simulink model "Sensor"  (R2022b)
settings: configuration reference "TmVcThermal_Configuration_sub" (kept outside this file)
undefined symbols (not defined in the file): cClCddSensor_t_u8AQSErrorConfirm, cClCddSensor_t_u8AQSErrorRelieve, cClCddSensor_Te_s32HvacEvapSensorOpenOrShortGnd, cClCddSensor_Te_s32HvacEvapSensorShortBatt, cClCddSensor_Te_s32HvacHexSensorOpenOrShortGnd, cClCddSensor_Te_s32HvacHexSensorShortBatt, cClCddSensor_Te_s32HvacIncarSensorOpenOrShortGnd, cClCddSensor_Te_s32HvacIncarSensorShortBatt, cClCddSensor_X_u8AQSErrorShape, cClCddSensor_X_u8AQSErrorShapeDevia, tClCddSensor_Te_s32EvapRtValue, tClCddSensor_Te_s32EvapRtValue_X, tClCddSensor_Te_s32HexRtValue, tClCddSensor_Te_s32HexRtValue_X, tClCddSensor_Te_s32IncarRtValue, tClCddSensor_Te_s32IncarRtValue_X
libraries: PCMULib x3, simulink x2
settings Model: PacingRate=0.500000  Creator=blue.ge  LastModifiedBy=blue.ge
settings ConfigSetRef: SourceName=TmVcThermal_Configuration_sub  SourceLocation=Base Workspace

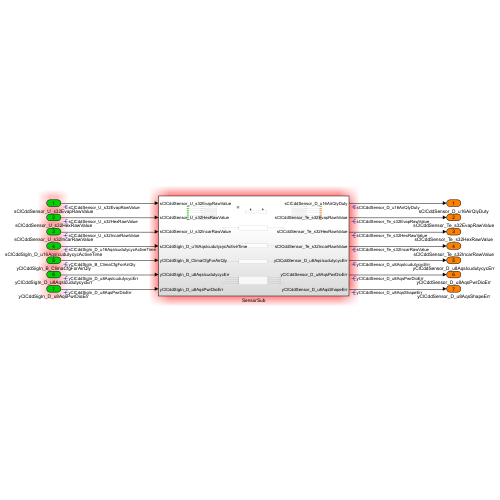
[thumbnail: Simulink's stored preview of the top-level diagram]
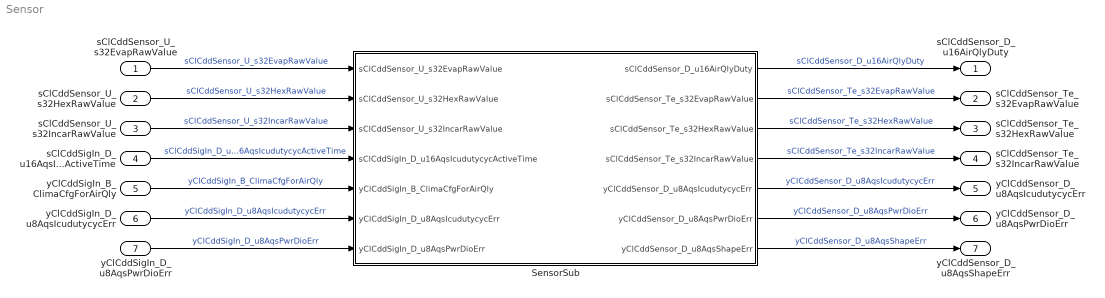
== system Sensor ==
  sClCddSensor_U_s32EvapRawValue : Inport  OutDataTypeStr=single
  sClCddSensor_U_s32HexRawValue : Inport  Port=2  OutDataTypeStr=single
  sClCddSensor_U_s32IncarRawValue : Inport  Port=3  OutDataTypeStr=single
  sClCddSigIn_D_u16AqsIcudutycycActiveTime : Inport  Port=4  OutDataTypeStr=uint16
  yClCddSigIn_B_ClimaCfgForAirQly : Inport  Port=5  OutDataTypeStr=boolean
  yClCddSigIn_D_u8AqsIcudutycycErr : Inport  Port=6  OutDataTypeStr=uint8
  yClCddSigIn_D_u8AqsPwrDioErr : Inport  Port=7  OutDataTypeStr=uint8
  SensorSub : Subsystem
  sClCddSensor_D_u16AirQlyDuty : Outport  OutDataTypeStr=uint16
  sClCddSensor_Te_s32EvapRawValue : Outport  Port=2  OutDataTypeStr=single
  sClCddSensor_Te_s32HexRawValue : Outport  Port=3  OutDataTypeStr=single
  sClCddSensor_Te_s32IncarRawValue : Outport  Port=4  OutDataTypeStr=single
  yClCddSensor_D_u8AqsIcudutycycErr : Outport  Port=5  OutDataTypeStr=uint8
  yClCddSensor_D_u8AqsPwrDioErr : Outport  Port=6  OutDataTypeStr=uint8
  yClCddSensor_D_u8AqsShapeErr : Outport  Port=7  OutDataTypeStr=uint8
  wires:
  SensorSub/5(yClCddSensor_D_u8AqsIcudutycycErr) -> yClCddSensor_D_u8AqsIcudutycycErr/1  "yClCddSensor_D_u8AqsIcudutycycErr"
  SensorSub/4(sClCddSensor_Te_s32IncarRawValue) -> sClCddSensor_Te_s32IncarRawValue/1  "sClCddSensor_Te_s32IncarRawValue"
  SensorSub/7(yClCddSensor_D_u8AqsShapeErr) -> yClCddSensor_D_u8AqsShapeErr/1  "yClCddSensor_D_u8AqsShapeErr"
  SensorSub/2(sClCddSensor_Te_s32EvapRawValue) -> sClCddSensor_Te_s32EvapRawValue/1  "sClCddSensor_Te_s32EvapRawValue"
  SensorSub/6(yClCddSensor_D_u8AqsPwrDioErr) -> yClCddSensor_D_u8AqsPwrDioErr/1  "yClCddSensor_D_u8AqsPwrDioErr"
  SensorSub/1(sClCddSensor_D_u16AirQlyDuty) -> sClCddSensor_D_u16AirQlyDuty/1  "sClCddSensor_D_u16AirQlyDuty"
  yClCddSigIn_D_u8AqsIcudutycycErr/1 -> SensorSub/6(yClCddSigIn_D_u8AqsIcudutycycErr)  "yClCddSigIn_D_u8AqsIcudutycycErr"
  sClCddSensor_U_s32EvapRawValue/1 -> SensorSub/1(sClCddSensor_U_s32EvapRawValue)  "sClCddSensor_U_s32EvapRawValue"
  sClCddSensor_U_s32IncarRawValue/1 -> SensorSub/3(sClCddSensor_U_s32IncarRawValue)  "sClCddSensor_U_s32IncarRawValue"
  yClCddSigIn_D_u8AqsPwrDioErr/1 -> SensorSub/7(yClCddSigIn_D_u8AqsPwrDioErr)  "yClCddSigIn_D_u8AqsPwrDioErr"
  sClCddSensor_U_s32HexRawValue/1 -> SensorSub/2(sClCddSensor_U_s32HexRawValue)  "sClCddSensor_U_s32HexRawValue"
  SensorSub/3(sClCddSensor_Te_s32HexRawValue) -> sClCddSensor_Te_s32HexRawValue/1  "sClCddSensor_Te_s32HexRawValue"
  yClCddSigIn_B_ClimaCfgForAirQly/1 -> SensorSub/5(yClCddSigIn_B_ClimaCfgForAirQly)  "yClCddSigIn_B_ClimaCfgForAirQly"
  sClCddSigIn_D_u16AqsIcudutycycActiveTime/1 -> SensorSub/4(sClCddSigIn_D_u16AqsIcudutycycActiveTime)  "sClCddSigIn_D_u16AqsIcudutycycActiveTime"

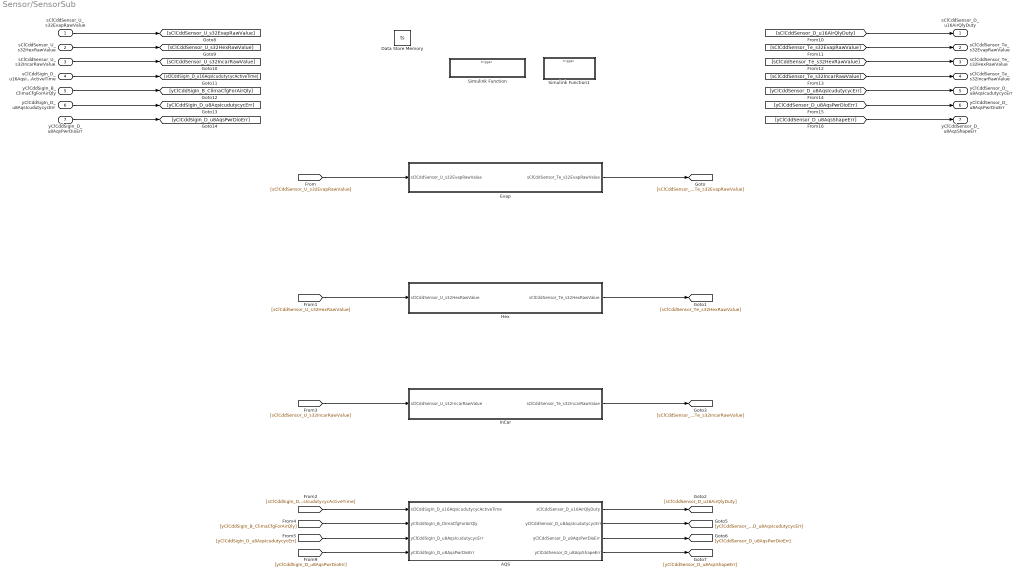
== system Sensor/SensorSub ==
  sClCddSensor_U_s32EvapRawValue : Inport  OutDataTypeStr=single
  sClCddSensor_U_s32HexRawValue : Inport  Port=2  OutDataTypeStr=single
  sClCddSensor_U_s32IncarRawValue : Inport  Port=3  OutDataTypeStr=single
  sClCddSigIn_D_u16AqsIcudutycycActiveTime : Inport  Port=4  OutDataTypeStr=uint16
  yClCddSigIn_B_ClimaCfgForAirQly : Inport  Port=5  OutDataTypeStr=boolean
  yClCddSigIn_D_u8AqsIcudutycycErr : Inport  Port=6  OutDataTypeStr=uint8
  yClCddSigIn_D_u8AqsPwrDioErr : Inport  Port=7  OutDataTypeStr=uint8
  AQS : Subsystem
  Data Store Memory : DataStoreMemory  DataStoreName=ts  ReadBeforeWriteMsg=warning  WriteAfterWriteMsg=warning  WriteAfterReadMsg=warning  InitialValue=0.05  ShowAdditionalParam=off  OutDataTypeStr=single
      settings: CopyFcn=set_param(gcbh,'ShowName','off');
  Evap : Subsystem
  Hex : Subsystem
  InCar : Subsystem
  Simulink Function : Subsystem  TreatAsAtomicUnit=on
  Simulink Function1 : Subsystem  TreatAsAtomicUnit=on
  sClCddSensor_D_u16AirQlyDuty : Outport  OutDataTypeStr=uint16
  sClCddSensor_Te_s32EvapRawValue : Outport  Port=2  OutDataTypeStr=single
  sClCddSensor_Te_s32HexRawValue : Outport  Port=3  OutDataTypeStr=single
  sClCddSensor_Te_s32IncarRawValue : Outport  Port=4  OutDataTypeStr=single
  yClCddSensor_D_u8AqsIcudutycycErr : Outport  Port=5  OutDataTypeStr=uint8
  yClCddSensor_D_u8AqsPwrDioErr : Outport  Port=6  OutDataTypeStr=uint8
  yClCddSensor_D_u8AqsShapeErr : Outport  Port=7  OutDataTypeStr=uint8
  wires:
  [sClCddSensor_U_s32EvapRawValue] -> Evap/1(sClCddSensor_U_s32EvapRawValue)
  Evap/1(sClCddSensor_Te_s32EvapRawValue) -> [sClCddSensor_Te_s32EvapRawValue]
  [sClCddSensor_U_s32HexRawValue] -> Hex/1(sClCddSensor_U_s32HexRawValue)
  Hex/1(sClCddSensor_Te_s32HexRawValue) -> [sClCddSensor_Te_s32HexRawValue]
  [sClCddSensor_U_s32IncarRawValue] -> InCar/1(sClCddSensor_U_s32IncarRawValue)
  InCar/1(sClCddSensor_Te_s32IncarRawValue) -> [sClCddSensor_Te_s32IncarRawValue]
  [sClCddSigIn_D_u16AqsIcudutycycActiveTime] -> AQS/1(sClCddSigIn_D_u16AqsIcudutycycActiveTime)
  [yClCddSigIn_B_ClimaCfgForAirQly] -> AQS/2(yClCddSigIn_B_ClimaCfgForAirQly)
  [yClCddSigIn_D_u8AqsIcudutycycErr] -> AQS/3(yClCddSigIn_D_u8AqsIcudutycycErr)
  [yClCddSigIn_D_u8AqsPwrDioErr] -> AQS/4(yClCddSigIn_D_u8AqsPwrDioErr)
  AQS/1(sClCddSensor_D_u16AirQlyDuty) -> [sClCddSensor_D_u16AirQlyDuty]
  AQS/2(yClCddSensor_D_u8AqsIcudutycycErr) -> [yClCddSensor_D_u8AqsIcudutycycErr]
  AQS/3(yClCddSensor_D_u8AqsPwrDioErr) -> [yClCddSensor_D_u8AqsPwrDioErr]
  AQS/4(yClCddSensor_D_u8AqsShapeErr) -> [yClCddSensor_D_u8AqsShapeErr]
  sClCddSensor_U_s32EvapRawValue/1 -> [sClCddSensor_U_s32EvapRawValue]
  sClCddSensor_U_s32HexRawValue/1 -> [sClCddSensor_U_s32HexRawValue]
  sClCddSensor_U_s32IncarRawValue/1 -> [sClCddSensor_U_s32IncarRawValue]
  sClCddSigIn_D_u16AqsIcudutycycActiveTime/1 -> [sClCddSigIn_D_u16AqsIcudutycycActiveTime]
  yClCddSigIn_B_ClimaCfgForAirQly/1 -> [yClCddSigIn_B_ClimaCfgForAirQly]
  yClCddSigIn_D_u8AqsIcudutycycErr/1 -> [yClCddSigIn_D_u8AqsIcudutycycErr]
  yClCddSigIn_D_u8AqsPwrDioErr/1 -> [yClCddSigIn_D_u8AqsPwrDioErr]
  [sClCddSensor_D_u16AirQlyDuty] -> sClCddSensor_D_u16AirQlyDuty/1
  [sClCddSensor_Te_s32EvapRawValue] -> sClCddSensor_Te_s32EvapRawValue/1
  [sClCddSensor_Te_s32HexRawValue] -> sClCddSensor_Te_s32HexRawValue/1
  [sClCddSensor_Te_s32IncarRawValue] -> sClCddSensor_Te_s32IncarRawValue/1
  [yClCddSensor_D_u8AqsIcudutycycErr] -> yClCddSensor_D_u8AqsIcudutycycErr/1
  [yClCddSensor_D_u8AqsPwrDioErr] -> yClCddSensor_D_u8AqsPwrDioErr/1
  [yClCddSensor_D_u8AqsShapeErr] -> yClCddSensor_D_u8AqsShapeErr/1

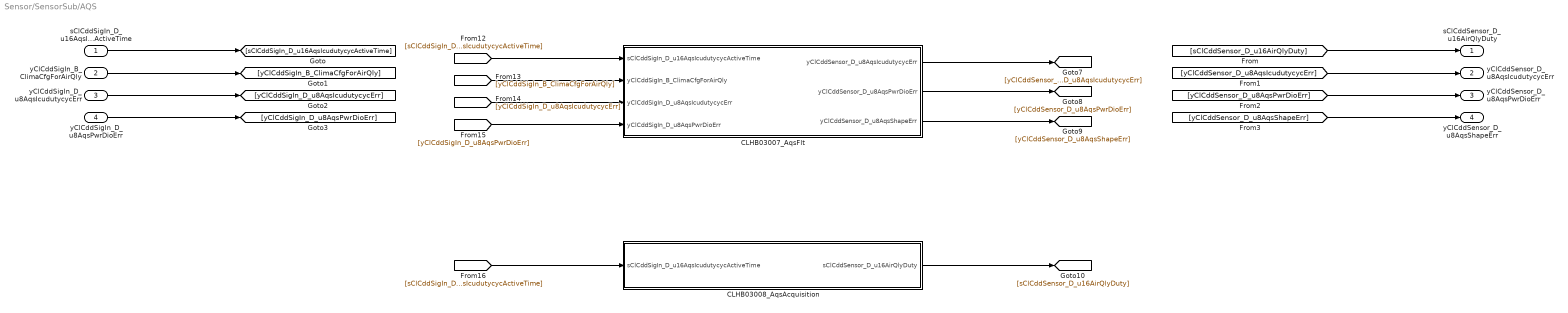
== system Sensor/SensorSub/AQS ==
  sClCddSigIn_D_u16AqsIcudutycycActiveTime : Inport  OutDataTypeStr=uint16
  yClCddSigIn_B_ClimaCfgForAirQly : Inport  Port=2  OutDataTypeStr=boolean
  yClCddSigIn_D_u8AqsIcudutycycErr : Inport  Port=3  OutDataTypeStr=uint8
  yClCddSigIn_D_u8AqsPwrDioErr : Inport  Port=4  OutDataTypeStr=uint8
  CLHB03007_AqsFlt : Subsystem
  CLHB03008_AqsAcquisition : Subsystem
  sClCddSensor_D_u16AirQlyDuty : Outport  OutDataTypeStr=uint16
  yClCddSensor_D_u8AqsIcudutycycErr : Outport  Port=2  OutDataTypeStr=uint8
  yClCddSensor_D_u8AqsPwrDioErr : Outport  Port=3  OutDataTypeStr=uint8
  yClCddSensor_D_u8AqsShapeErr : Outport  Port=4  OutDataTypeStr=uint8
  wires:
  [yClCddSigIn_D_u8AqsIcudutycycErr] -> CLHB03007_AqsFlt/3(yClCddSigIn_D_u8AqsIcudutycycErr)
  [sClCddSigIn_D_u16AqsIcudutycycActiveTime] -> CLHB03008_AqsAcquisition/1(sClCddSigIn_D_u16AqsIcudutycycActiveTime)
  CLHB03007_AqsFlt/2(yClCddSensor_D_u8AqsPwrDioErr) -> [yClCddSensor_D_u8AqsPwrDioErr]
  CLHB03007_AqsFlt/1(yClCddSensor_D_u8AqsIcudutycycErr) -> [yClCddSensor_D_u8AqsIcudutycycErr]
  [sClCddSigIn_D_u16AqsIcudutycycActiveTime] -> CLHB03007_AqsFlt/1(sClCddSigIn_D_u16AqsIcudutycycActiveTime)
  CLHB03008_AqsAcquisition/1(sClCddSensor_D_u16AirQlyDuty) -> [sClCddSensor_D_u16AirQlyDuty]
  [yClCddSigIn_B_ClimaCfgForAirQly] -> CLHB03007_AqsFlt/2(yClCddSigIn_B_ClimaCfgForAirQly)
  CLHB03007_AqsFlt/3(yClCddSensor_D_u8AqsShapeErr) -> [yClCddSensor_D_u8AqsShapeErr]
  [yClCddSigIn_D_u8AqsPwrDioErr] -> CLHB03007_AqsFlt/4(yClCddSigIn_D_u8AqsPwrDioErr)
  sClCddSigIn_D_u16AqsIcudutycycActiveTime/1 -> [sClCddSigIn_D_u16AqsIcudutycycActiveTime]
  yClCddSigIn_B_ClimaCfgForAirQly/1 -> [yClCddSigIn_B_ClimaCfgForAirQly]
  yClCddSigIn_D_u8AqsIcudutycycErr/1 -> [yClCddSigIn_D_u8AqsIcudutycycErr]
  yClCddSigIn_D_u8AqsPwrDioErr/1 -> [yClCddSigIn_D_u8AqsPwrDioErr]
  [sClCddSensor_D_u16AirQlyDuty] -> sClCddSensor_D_u16AirQlyDuty/1
  [yClCddSensor_D_u8AqsIcudutycycErr] -> yClCddSensor_D_u8AqsIcudutycycErr/1
  [yClCddSensor_D_u8AqsPwrDioErr] -> yClCddSensor_D_u8AqsPwrDioErr/1
  [yClCddSensor_D_u8AqsShapeErr] -> yClCddSensor_D_u8AqsShapeErr/1

== system Sensor/SensorSub/Evap ==
  sClCddSensor_U_s32EvapRawValue : Inport  OutDataTypeStr=single
  CLHB03002_EvapChange : Subsystem
  CLHB03002_EvapFlt : Subsystem
  sClCddSensor_Te_s32EvapRawValue : Outport  OutDataTypeStr=single
  wires:
  [sClCddSensor_U_s32EvapRawValue] -> CLHB03002_EvapFlt/1(sClCddSensor_U_s32EvapRawValue)
  [sClCddSensor_D_u8HvacEvapSensorErr] -> CLHB03002_EvapChange/2(sClCddSensor_D_u8HvacEvapSensorErr)
  CLHB03002_EvapChange/1(sClCddSensor_Te_s32EvapRawValue) -> [sClCddSensor_Te_s32EvapRawValue]
  CLHB03002_EvapFlt/1(sClCddSensor_D_u8HvacEvapSensorErr) -> [sClCddSensor_D_u8HvacEvapSensorErr]
  [sClCddSensor_U_s32EvapRawValue] -> CLHB03002_EvapChange/1(sClCddSensor_U_s32EvapRawValue)
  sClCddSensor_U_s32EvapRawValue/1 -> [sClCddSensor_U_s32EvapRawValue]
  [sClCddSensor_Te_s32EvapRawValue] -> sClCddSensor_Te_s32EvapRawValue/1

== system Sensor/SensorSub/Hex ==
  sClCddSensor_U_s32HexRawValue : Inport  OutDataTypeStr=single
  CLHB03003_HexFlt : Subsystem
  CLHB03004_HexChange : Subsystem
  sClCddSensor_Te_s32HexRawValue : Outport  OutDataTypeStr=single
  wires:
  [sClCddSensor_U_s32HexRawValue] -> CLHB03003_HexFlt/1(sClCddSensor_U_s32HexRawValue)
  CLHB03003_HexFlt/1(sClCddSensor_D_u8HvacHexSensorErr) -> [sClCddSensor_D_u8HvacHexSensorErr]
  [sClCddSensor_U_s32HexRawValue] -> CLHB03004_HexChange/1("sClCddSensor_U_s32HexRawValue ")
  [sClCddSensor_D_u8HvacHexSensorErr] -> CLHB03004_HexChange/2("sClCddSensor_D_u8HvacHexSensorErr ")
  CLHB03004_HexChange/1("sClCddSensor_Te_s32HexRawValue ") -> [sClCddSensor_Te_s32HexRawValue]
  sClCddSensor_U_s32HexRawValue/1 -> [sClCddSensor_U_s32HexRawValue]
  [sClCddSensor_Te_s32HexRawValue] -> sClCddSensor_Te_s32HexRawValue/1

== system Sensor/SensorSub/InCar ==
  sClCddSensor_U_s32IncarRawValue : Inport  OutDataTypeStr=single
  CLHB03005_InCarFlt : Subsystem
  CLHB03006_InCarChange : Subsystem
  sClCddSensor_Te_s32IncarRawValue : Outport  OutDataTypeStr=single
  wires:
  CLHB03006_InCarChange/1(sClCddSensor_Te_s32IncarRawValue) -> [sClCddSensor_Te_s32IncarRawValue]
  [sClCddSensor_U_s32IncarRawValue] -> CLHB03005_InCarFlt/1(sClCddSensor_U_s32IncarRawValue)
  CLHB03005_InCarFlt/1(sClCddSensor_D_u8HvacIncarSensorErr) -> [sClCddSensor_D_u8HvacIncarSensorErr]
  [sClCddSensor_D_u8HvacIncarSensorErr] -> CLHB03006_InCarChange/1(sClCddSensor_D_u8HvacIncarSensorErr)
  [sClCddSensor_U_s32IncarRawValue] -> CLHB03006_InCarChange/2(sClCddSensor_U_s32IncarRawValue)
  sClCddSensor_U_s32IncarRawValue/1 -> [sClCddSensor_U_s32IncarRawValue]
  [sClCddSensor_Te_s32IncarRawValue] -> sClCddSensor_Te_s32IncarRawValue/1

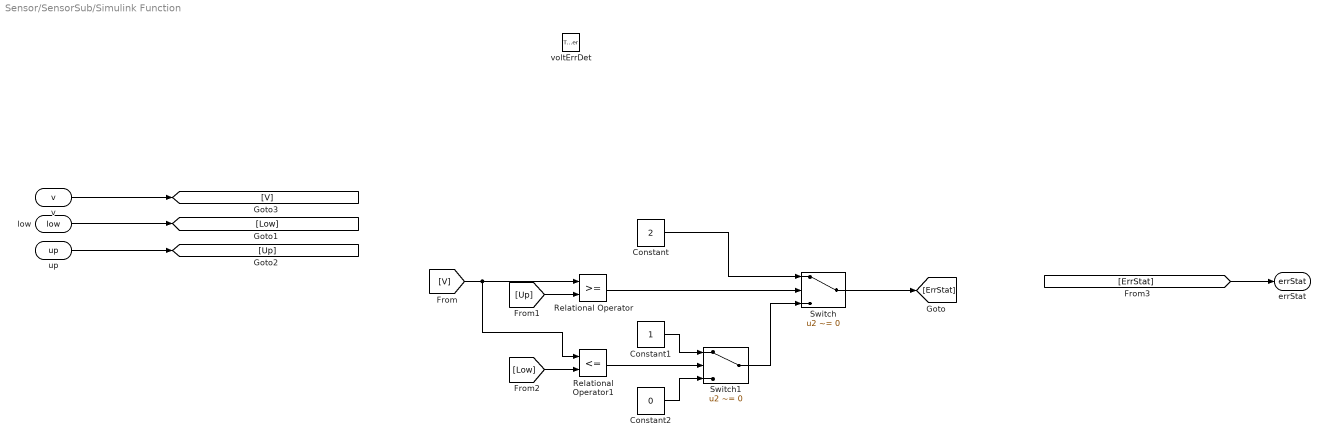
== system Sensor/SensorSub/Simulink Function ==
  voltErrDet : TriggerPort  TriggerType=function-call  IsSimulinkFunction=on  FunctionName=voltErrDet  FunctionVisibility=scoped  VariantControl=(inherit)
  Constant : Constant  Value=2  OutDataTypeStr=uint8
  Constant1 : Constant  OutDataTypeStr=uint8
  Constant2 : Constant  Value=0  OutDataTypeStr=uint8
  Relational Operator : RelationalOperator  OutDataTypeStr=boolean  RndMeth=Simplest  InputSameDT=off
  Relational Operator1 : RelationalOperator  Operator=<=  OutDataTypeStr=boolean  RndMeth=Simplest  InputSameDT=off
  Switch : Switch  Criteria=u2 ~= 0  OutDataTypeStr=uint8  SaturateOnIntegerOverflow=off  InputSameDT=off
  Switch1 : Switch  Criteria=u2 ~= 0  OutDataTypeStr=uint8  SaturateOnIntegerOverflow=off  InputSameDT=off
  v : ArgIn  DisableCoverage=on  OutDataTypeStr=single  ArgumentName=v
  low : ArgIn  DisableCoverage=on  Port=2  OutDataTypeStr=single  ArgumentName=low
  up : ArgIn  DisableCoverage=on  Port=3  OutDataTypeStr=single  ArgumentName=up
  errStat : ArgOut  DisableCoverage=on  OutDataTypeStr=uint8  ArgumentName=errStat
  wires:
  [V] -> Relational Operator1/1, Relational Operator/1
  Switch1/1 -> Switch/3
  Constant1/1 -> Switch1/1
  [Low] -> Relational Operator1/2
  Relational Operator/1 -> Switch/2
  Switch/1 -> [ErrStat]
  Relational Operator1/1 -> Switch1/2
  Constant/1 -> Switch/1
  [Up] -> Relational Operator/2
  Constant2/1 -> Switch1/3
  low/1 -> [Low]
  up/1 -> [Up]
  v/1 -> [V]
  [ErrStat] -> errStat/1

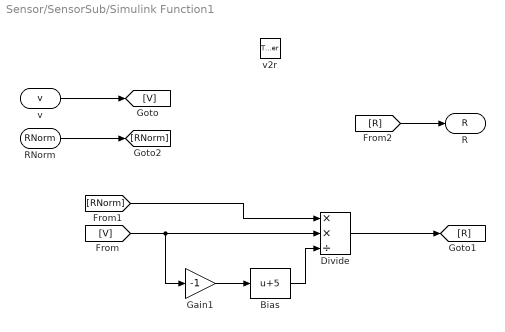
== system Sensor/SensorSub/Simulink Function1 ==
  v2r : TriggerPort  TriggerType=function-call  IsSimulinkFunction=on  FunctionName=v2r  FunctionVisibility=scoped  VariantControl=(inherit)
  Bias : Bias  Bias=5  SaturateOnIntegerOverflow=off
  Divide : Product  Inputs=**/
  Gain1 : Gain  Gain=-1
  v : ArgIn  DisableCoverage=on  OutDataTypeStr=single  ArgumentName=v
  RNorm : ArgIn  DisableCoverage=on  Port=2  OutDataTypeStr=single  ArgumentName=RNorm
  R : ArgOut  DisableCoverage=on  OutDataTypeStr=single  ArgumentName=R
  wires:
  [V] -> Divide/2, Gain1/1
  Gain1/1 -> Bias/1
  Divide/1 -> [R]
  v/1 -> [V]
  RNorm/1 -> [RNorm]
  Bias/1 -> Divide/3
  [RNorm] -> Divide/1
  [R] -> R/1

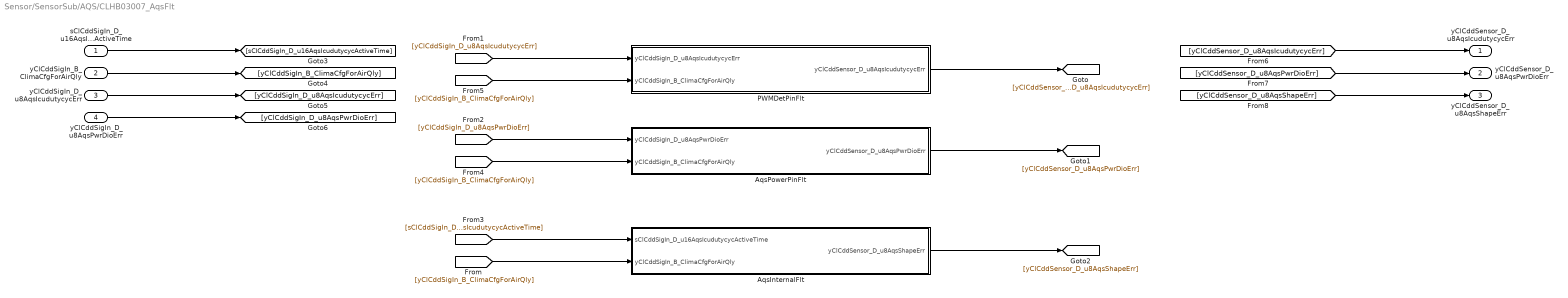
== system Sensor/SensorSub/AQS/CLHB03007_AqsFlt ==
  sClCddSigIn_D_u16AqsIcudutycycActiveTime : Inport  OutDataTypeStr=uint16
  yClCddSigIn_B_ClimaCfgForAirQly : Inport  Port=2  OutDataTypeStr=boolean
  yClCddSigIn_D_u8AqsIcudutycycErr : Inport  Port=3  OutDataTypeStr=uint8
  yClCddSigIn_D_u8AqsPwrDioErr : Inport  Port=4  OutDataTypeStr=uint8
  AqsInternalFlt : Subsystem
  AqsPowerPinFlt : Subsystem
  PWMDetPinFlt : Subsystem
  yClCddSensor_D_u8AqsIcudutycycErr : Outport  OutDataTypeStr=uint8
  yClCddSensor_D_u8AqsPwrDioErr : Outport  Port=2  OutDataTypeStr=uint8
  yClCddSensor_D_u8AqsShapeErr : Outport  Port=3  OutDataTypeStr=uint8
  wires:
  [yClCddSigIn_D_u8AqsIcudutycycErr] -> PWMDetPinFlt/1(yClCddSigIn_D_u8AqsIcudutycycErr)
  PWMDetPinFlt/1(yClCddSensor_D_u8AqsIcudutycycErr) -> [yClCddSensor_D_u8AqsIcudutycycErr]
  [yClCddSigIn_D_u8AqsPwrDioErr] -> AqsPowerPinFlt/1(yClCddSigIn_D_u8AqsPwrDioErr)
  AqsPowerPinFlt/1(yClCddSensor_D_u8AqsPwrDioErr) -> [yClCddSensor_D_u8AqsPwrDioErr]
  [sClCddSigIn_D_u16AqsIcudutycycActiveTime] -> AqsInternalFlt/1(sClCddSigIn_D_u16AqsIcudutycycActiveTime)
  AqsInternalFlt/1(yClCddSensor_D_u8AqsShapeErr) -> [yClCddSensor_D_u8AqsShapeErr]
  [yClCddSigIn_B_ClimaCfgForAirQly] -> AqsInternalFlt/2(yClCddSigIn_B_ClimaCfgForAirQly)
  [yClCddSigIn_B_ClimaCfgForAirQly] -> AqsPowerPinFlt/2(yClCddSigIn_B_ClimaCfgForAirQly)
  [yClCddSigIn_B_ClimaCfgForAirQly] -> PWMDetPinFlt/2(yClCddSigIn_B_ClimaCfgForAirQly)
  sClCddSigIn_D_u16AqsIcudutycycActiveTime/1 -> [sClCddSigIn_D_u16AqsIcudutycycActiveTime]
  yClCddSigIn_B_ClimaCfgForAirQly/1 -> [yClCddSigIn_B_ClimaCfgForAirQly]
  yClCddSigIn_D_u8AqsIcudutycycErr/1 -> [yClCddSigIn_D_u8AqsIcudutycycErr]
  yClCddSigIn_D_u8AqsPwrDioErr/1 -> [yClCddSigIn_D_u8AqsPwrDioErr]
  [yClCddSensor_D_u8AqsIcudutycycErr] -> yClCddSensor_D_u8AqsIcudutycycErr/1
  [yClCddSensor_D_u8AqsPwrDioErr] -> yClCddSensor_D_u8AqsPwrDioErr/1
  [yClCddSensor_D_u8AqsShapeErr] -> yClCddSensor_D_u8AqsShapeErr/1

== system Sensor/SensorSub/AQS/CLHB03008_AqsAcquisition ==
  sClCddSigIn_D_u16AqsIcudutycycActiveTime : Inport  OutDataTypeStr=uint16
  Gain : Gain  Gain=10  OutDataTypeStr=uint16
  sClCddSensor_D_u16AirQlyDuty : Outport  OutDataTypeStr=uint16
  wires:
  [sClCddSigIn_D_u16AqsIcudutycycActiveTime] -> Gain/1
  Gain/1 -> [sClCddSensor_D_u16AirQlyDuty]
  sClCddSigIn_D_u16AqsIcudutycycActiveTime/1 -> [sClCddSigIn_D_u16AqsIcudutycycActiveTime]
  [sClCddSensor_D_u16AirQlyDuty] -> sClCddSensor_D_u16AirQlyDuty/1

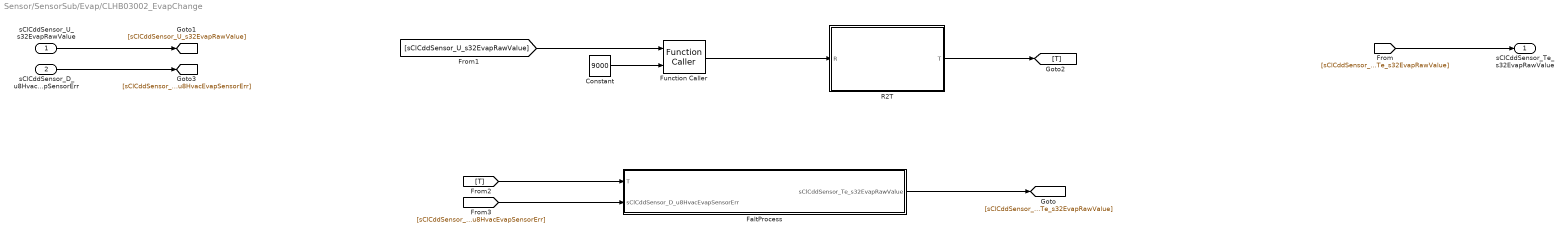
== system Sensor/SensorSub/Evap/CLHB03002_EvapChange ==
  sClCddSensor_U_s32EvapRawValue : Inport  OutDataTypeStr=single
  sClCddSensor_D_u8HvacEvapSensorErr : Inport  Port=2  OutDataTypeStr=uint8
  Constant : Constant  Value=9000  OutDataTypeStr=single
  FaltProcess : Subsystem
  Function Caller : FunctionCaller  FunctionPrototype=R = v2r(v,RNorm)  InputArgumentSpecifications=<Enter example>  OutputArgumentSpecifications=<Enter example>
  R2T : Subsystem
  sClCddSensor_Te_s32EvapRawValue : Outport  OutDataTypeStr=single
  wires:
  Function Caller/1 -> R2T/1(R)
  sClCddSensor_U_s32EvapRawValue/1 -> [sClCddSensor_U_s32EvapRawValue]
  [sClCddSensor_Te_s32EvapRawValue] -> sClCddSensor_Te_s32EvapRawValue/1
  R2T/1(T) -> [T]
  [T] -> FaltProcess/1(T)
  [sClCddSensor_D_u8HvacEvapSensorErr] -> FaltProcess/2(sClCddSensor_D_u8HvacEvapSensorErr)
  FaltProcess/1(sClCddSensor_Te_s32EvapRawValue) -> [sClCddSensor_Te_s32EvapRawValue]
  sClCddSensor_D_u8HvacEvapSensorErr/1 -> [sClCddSensor_D_u8HvacEvapSensorErr]
  Constant/1 -> Function Caller/2
  [sClCddSensor_U_s32EvapRawValue] -> Function Caller/1

== system Sensor/SensorSub/Evap/CLHB03002_EvapFlt ==
  sClCddSensor_U_s32EvapRawValue : Inport  OutDataTypeStr=single
  Constant3 : Constant  Value=cClCddSensor_Te_s32HvacEvapSensorOpenOrShortGnd  OutDataTypeStr=single
  Constant4 : Constant  Value=cClCddSensor_Te_s32HvacEvapSensorShortBatt  OutDataTypeStr=single
  Function Caller : FunctionCaller  FunctionPrototype=errStat = voltErrDet(v,low,up)  InputArgumentSpecifications=<Enter example>  OutputArgumentSpecifications=<Enter example>
  sClCddSensor_D_u8HvacEvapSensorErr : Outport  OutDataTypeStr=uint8
  wires:
  sClCddSensor_U_s32EvapRawValue/1 -> [sClCddSensor_U_s32EvapRawValue]
  [sClCddSensor_D_u8HvacEvapSensorErr] -> sClCddSensor_D_u8HvacEvapSensorErr/1
  Constant3/1 -> Function Caller/2
  Constant4/1 -> Function Caller/3
  [sClCddSensor_U_s32EvapRawValue] -> Function Caller/1
  Function Caller/1 -> [sClCddSensor_D_u8HvacEvapSensorErr]

== system Sensor/SensorSub/Hex/CLHB03003_HexFlt ==
  sClCddSensor_U_s32HexRawValue : Inport  OutDataTypeStr=single
  Constant3 : Constant  Value=cClCddSensor_Te_s32HvacHexSensorOpenOrShortGnd  OutDataTypeStr=single
  Constant4 : Constant  Value=cClCddSensor_Te_s32HvacHexSensorShortBatt  OutDataTypeStr=single
  Function Caller : FunctionCaller  FunctionPrototype=errStat = voltErrDet(v,low,up)  InputArgumentSpecifications=<Enter example>  OutputArgumentSpecifications=<Enter example>
  sClCddSensor_D_u8HvacHexSensorErr : Outport  OutDataTypeStr=uint8
  wires:
  [sClCddSensor_D_u8HvacHexSensorErr] -> sClCddSensor_D_u8HvacHexSensorErr/1
  sClCddSensor_U_s32HexRawValue/1 -> [sClCddSensor_U_s32HexRawValue]
  [sClCddSensor_U_s32HexRawValue] -> Function Caller/1
  Function Caller/1 -> [sClCddSensor_D_u8HvacHexSensorErr]
  Constant3/1 -> Function Caller/2
  Constant4/1 -> Function Caller/3

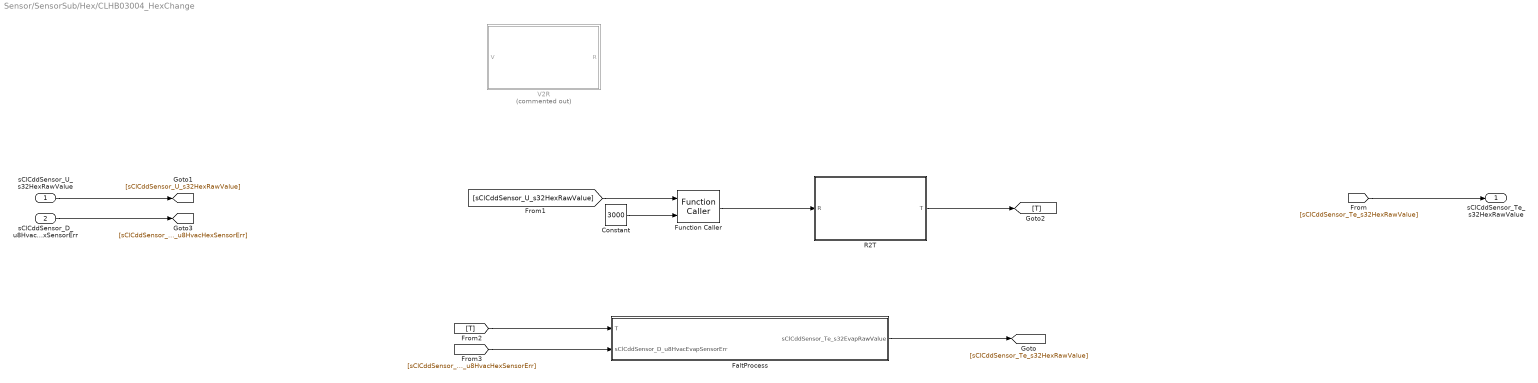
== system Sensor/SensorSub/Hex/CLHB03004_HexChange ==
  "sClCddSensor_U_s32HexRawValue " : Inport  OutDataTypeStr=single
  "sClCddSensor_D_u8HvacHexSensorErr " : Inport  Port=2  OutDataTypeStr=uint8
  Constant : Constant  Value=3000  OutDataTypeStr=single
  FaltProcess : Subsystem
  Function Caller : FunctionCaller  FunctionPrototype=R = v2r(v,RNorm)  InputArgumentSpecifications=<Enter example>  OutputArgumentSpecifications=<Enter example>
  R2T : Subsystem
  V2R : Subsystem  Commented=on
  "sClCddSensor_Te_s32HexRawValue " : Outport  OutDataTypeStr=single
  wires:
  FaltProcess/1(sClCddSensor_Te_s32EvapRawValue) -> [sClCddSensor_Te_s32HexRawValue]
  [sClCddSensor_Te_s32HexRawValue] -> "sClCddSensor_Te_s32HexRawValue "/1
  "sClCddSensor_D_u8HvacHexSensorErr "/1 -> [sClCddSensor_D_u8HvacHexSensorErr]
  [T] -> FaltProcess/1(T)
  [sClCddSensor_D_u8HvacHexSensorErr] -> FaltProcess/2(sClCddSensor_D_u8HvacEvapSensorErr)
  R2T/1(T) -> [T]
  "sClCddSensor_U_s32HexRawValue "/1 -> [sClCddSensor_U_s32HexRawValue]
  Constant/1 -> Function Caller/2
  [sClCddSensor_U_s32HexRawValue] -> Function Caller/1
  Function Caller/1 -> R2T/1(R)

== system Sensor/SensorSub/InCar/CLHB03005_InCarFlt ==
  sClCddSensor_U_s32IncarRawValue : Inport  OutDataTypeStr=single
  Constant : Constant  Value=cClCddSensor_Te_s32HvacIncarSensorOpenOrShortGnd  OutDataTypeStr=single
  Constant1 : Constant  Value=cClCddSensor_Te_s32HvacIncarSensorShortBatt  OutDataTypeStr=single
  Function Caller : FunctionCaller  FunctionPrototype=errStat = voltErrDet(v,low,up)  InputArgumentSpecifications=<Enter example>  OutputArgumentSpecifications=<Enter example>
  sClCddSensor_D_u8HvacIncarSensorErr : Outport  OutDataTypeStr=uint8
  wires:
  [sClCddSensor_U_s32IncarRawValue] -> Function Caller/1
  Constant/1 -> Function Caller/2
  Constant1/1 -> Function Caller/3
  Function Caller/1 -> [sClCddSensor_D_u8HvacIncarSensorErr]
  sClCddSensor_U_s32IncarRawValue/1 -> [sClCddSensor_U_s32IncarRawValue]
  [sClCddSensor_D_u8HvacIncarSensorErr] -> sClCddSensor_D_u8HvacIncarSensorErr/1

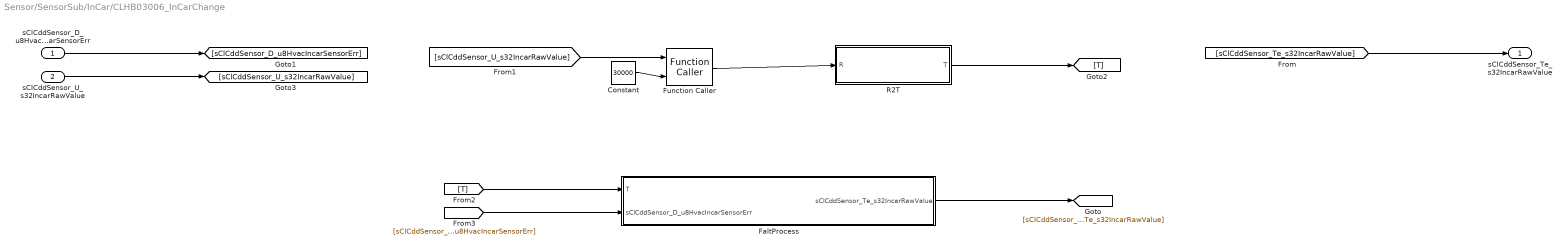
== system Sensor/SensorSub/InCar/CLHB03006_InCarChange ==
  sClCddSensor_D_u8HvacIncarSensorErr : Inport  OutDataTypeStr=uint8
  sClCddSensor_U_s32IncarRawValue : Inport  Port=2  OutDataTypeStr=single
  Constant : Constant  Value=30000  OutDataTypeStr=single
  FaltProcess : Subsystem
  Function Caller : FunctionCaller  FunctionPrototype=R = v2r(v,RNorm)  InputArgumentSpecifications=<Enter example>  OutputArgumentSpecifications=<Enter example>
  R2T : Subsystem
  sClCddSensor_Te_s32IncarRawValue : Outport  OutDataTypeStr=single
  wires:
  R2T/1(T) -> [T]
  [sClCddSensor_D_u8HvacIncarSensorErr] -> FaltProcess/2("sClCddSensor_D_u8HvacIncarSensorErr  ")
  [T] -> FaltProcess/1(T)
  FaltProcess/1(sClCddSensor_Te_s32IncarRawValue) -> [sClCddSensor_Te_s32IncarRawValue]
  [sClCddSensor_U_s32IncarRawValue] -> Function Caller/1
  Constant/1 -> Function Caller/2
  Function Caller/1 -> R2T/1(R)
  sClCddSensor_D_u8HvacIncarSensorErr/1 -> [sClCddSensor_D_u8HvacIncarSensorErr]
  sClCddSensor_U_s32IncarRawValue/1 -> [sClCddSensor_U_s32IncarRawValue]
  [sClCddSensor_Te_s32IncarRawValue] -> sClCddSensor_Te_s32IncarRawValue/1

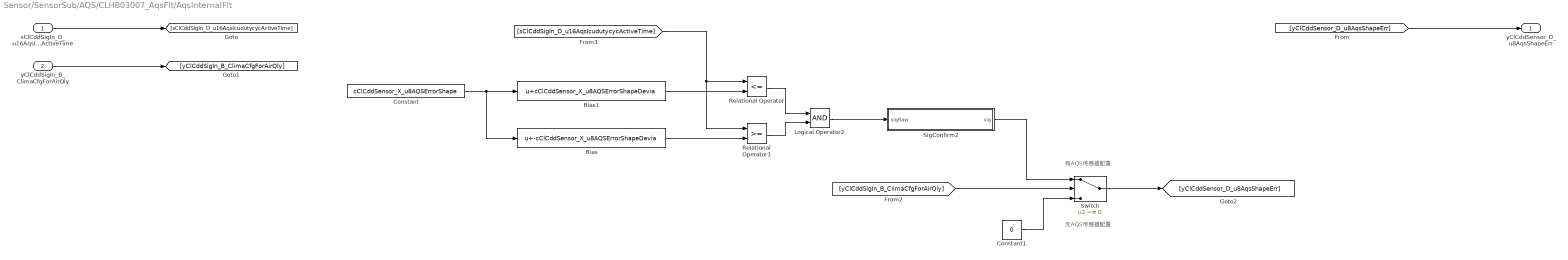
== system Sensor/SensorSub/AQS/CLHB03007_AqsFlt/AqsInternalFlt ==
  note: 有AQS传感器配置
  note: 无AQS传感器配置
  sClCddSigIn_D_u16AqsIcudutycycActiveTime : Inport  OutDataTypeStr=uint16
  yClCddSigIn_B_ClimaCfgForAirQly : Inport  Port=2  OutDataTypeStr=boolean
  Bias : Bias  Bias=-cClCddSensor_X_u8AQSErrorShapeDevia  SaturateOnIntegerOverflow=off
  Bias1 : Bias  Bias=cClCddSensor_X_u8AQSErrorShapeDevia  SaturateOnIntegerOverflow=off
  Constant : Constant  Value=cClCddSensor_X_u8AQSErrorShape  OutDataTypeStr=uint8
  Constant1 : Constant  Value=0  OutDataTypeStr=uint8
  Logical Operator2 : Logic  AllPortsSameDT=off  OutDataTypeStr=boolean
  Relational Operator : RelationalOperator  Operator=<=  OutDataTypeStr=boolean  RndMeth=Simplest  InputSameDT=off
  Relational Operator1 : RelationalOperator  OutDataTypeStr=boolean  RndMeth=Simplest  InputSameDT=off
  SigConfirm2 : Subsystem
  Switch : Switch  Criteria=u2 ~= 0  SaturateOnIntegerOverflow=off  InputSameDT=off
  yClCddSensor_D_u8AqsShapeErr : Outport  OutDataTypeStr=uint8
  wires:
  Constant/1 -> Bias/1, Bias1/1
  Relational Operator/1 -> Logical Operator2/1
  Bias/1 -> Relational Operator1/2
  [sClCddSigIn_D_u16AqsIcudutycycActiveTime] -> Relational Operator1/1, Relational Operator/1
  Bias1/1 -> Relational Operator/2
  Logical Operator2/1 -> SigConfirm2/1(sigRaw)
  Relational Operator1/1 -> Logical Operator2/2
  sClCddSigIn_D_u16AqsIcudutycycActiveTime/1 -> [sClCddSigIn_D_u16AqsIcudutycycActiveTime]
  [yClCddSensor_D_u8AqsShapeErr] -> yClCddSensor_D_u8AqsShapeErr/1
  [yClCddSigIn_B_ClimaCfgForAirQly] -> Switch/2
  SigConfirm2/1(sig) -> Switch/1
  Constant1/1 -> Switch/3
  Switch/1 -> [yClCddSensor_D_u8AqsShapeErr]
  yClCddSigIn_B_ClimaCfgForAirQly/1 -> [yClCddSigIn_B_ClimaCfgForAirQly]

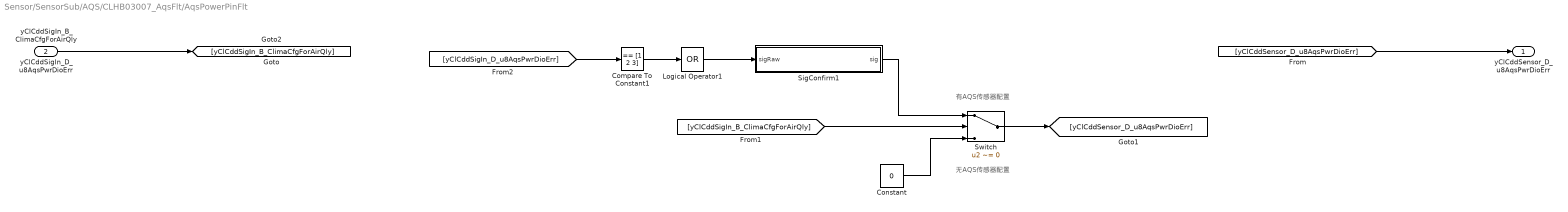
== system Sensor/SensorSub/AQS/CLHB03007_AqsFlt/AqsPowerPinFlt ==
  note: 有AQS传感器配置
  note: 无AQS传感器配置
  yClCddSigIn_D_u8AqsPwrDioErr : Inport  OutDataTypeStr=uint8
  yClCddSigIn_B_ClimaCfgForAirQly : Inport  Port=2  OutDataTypeStr=boolean
  Compare To Constant1 : simulink/Logic and Bit Operations/Compare To Constant  relop===  const=[1 2 3]  OutDataTypeStr=boolean
  Constant : Constant  Value=0  OutDataTypeStr=uint8
  Logical Operator1 : Logic  Operator=OR  Inputs=1  AllPortsSameDT=off  OutDataTypeStr=boolean
  SigConfirm1 : Subsystem
  Switch : Switch  Criteria=u2 ~= 0  SaturateOnIntegerOverflow=off  InputSameDT=off
  yClCddSensor_D_u8AqsPwrDioErr : Outport  OutDataTypeStr=uint8
  wires:
  [yClCddSigIn_D_u8AqsPwrDioErr] -> Compare To Constant1/1
  Compare To Constant1/1 -> Logical Operator1/1
  Logical Operator1/1 -> SigConfirm1/1(sigRaw)
  yClCddSigIn_D_u8AqsPwrDioErr/1 -> [yClCddSigIn_D_u8AqsPwrDioErr]
  [yClCddSensor_D_u8AqsPwrDioErr] -> yClCddSensor_D_u8AqsPwrDioErr/1
  [yClCddSigIn_B_ClimaCfgForAirQly] -> Switch/2
  SigConfirm1/1(sig) -> Switch/1
  Constant/1 -> Switch/3
  Switch/1 -> [yClCddSensor_D_u8AqsPwrDioErr]
  yClCddSigIn_B_ClimaCfgForAirQly/1 -> [yClCddSigIn_B_ClimaCfgForAirQly]

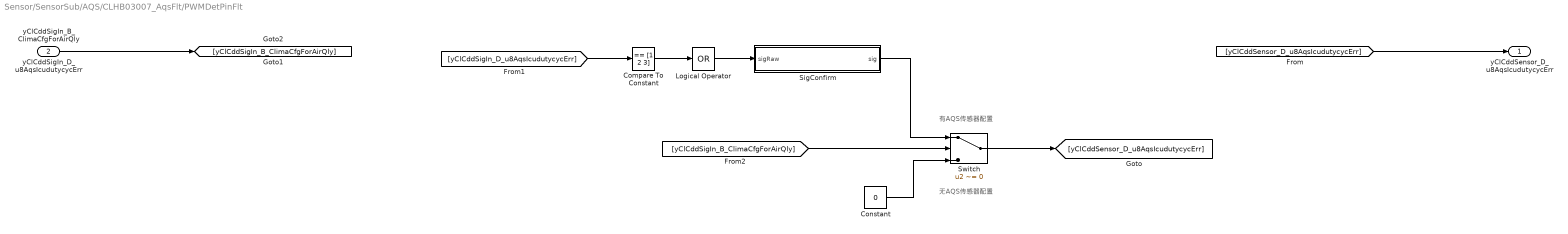
== system Sensor/SensorSub/AQS/CLHB03007_AqsFlt/PWMDetPinFlt ==
  note: 无AQS传感器配置
  note: 有AQS传感器配置
  yClCddSigIn_D_u8AqsIcudutycycErr : Inport  OutDataTypeStr=uint8
  yClCddSigIn_B_ClimaCfgForAirQly : Inport  Port=2  OutDataTypeStr=boolean
  Compare To Constant : simulink/Logic and Bit Operations/Compare To Constant  relop===  const=[1 2 3]  OutDataTypeStr=boolean
  Constant : Constant  Value=0  OutDataTypeStr=uint8
  Logical Operator : Logic  Operator=OR  Inputs=1  AllPortsSameDT=off  OutDataTypeStr=boolean
  SigConfirm : Subsystem
  Switch : Switch  Criteria=u2 ~= 0  SaturateOnIntegerOverflow=off  InputSameDT=off
  yClCddSensor_D_u8AqsIcudutycycErr : Outport  OutDataTypeStr=uint8
  wires:
  Logical Operator/1 -> SigConfirm/1(sigRaw)
  Compare To Constant/1 -> Logical Operator/1
  [yClCddSigIn_D_u8AqsIcudutycycErr] -> Compare To Constant/1
  yClCddSigIn_D_u8AqsIcudutycycErr/1 -> [yClCddSigIn_D_u8AqsIcudutycycErr]
  [yClCddSensor_D_u8AqsIcudutycycErr] -> yClCddSensor_D_u8AqsIcudutycycErr/1
  [yClCddSigIn_B_ClimaCfgForAirQly] -> Switch/2
  Switch/1 -> [yClCddSensor_D_u8AqsIcudutycycErr]
  SigConfirm/1(sig) -> Switch/1
  Constant/1 -> Switch/3
  yClCddSigIn_B_ClimaCfgForAirQly/1 -> [yClCddSigIn_B_ClimaCfgForAirQly]

== system Sensor/SensorSub/Evap/CLHB03002_EvapChange/FaltProcess ==
  T : Inport
  sClCddSensor_D_u8HvacEvapSensorErr : Inport  Port=2  OutDataTypeStr=uint8
  Switch : Switch  Criteria=u2 ~= 0  OutDataTypeStr=single  SaturateOnIntegerOverflow=off  InputSameDT=off
  Unit Delay : UnitDelay  SampleTime=-1  HasFrameUpgradeWarning=on
  sClCddSensor_Te_s32EvapRawValue : Outport  OutDataTypeStr=single
  wires:
  Unit Delay/1 -> Switch/1
  Switch/1 -> [sClCddSensor_Te_s32EvapRawValue], Unit Delay/1
  [T] -> Switch/3
  [sClCddSensor_D_u8HvacEvapSensorErr] -> Switch/2
  T/1 -> [T]
  sClCddSensor_D_u8HvacEvapSensorErr/1 -> [sClCddSensor_D_u8HvacEvapSensorErr]
  [sClCddSensor_Te_s32EvapRawValue] -> sClCddSensor_Te_s32EvapRawValue/1

== system Sensor/SensorSub/Evap/CLHB03002_EvapChange/R2T ==
  R : Inport
  1-D Lookup Table : Lookup_n-D  NumberOfTableDimensions=1  BreakpointsForDimension1=tClCddSensor_Te_s32EvapRtValue_X  BreakpointsForDimension1DataTypeStr=Inherit: Inherit from 'Breakpoint data'  Table=tClCddSensor_Te_s32EvapRtValue  TableDataTypeStr=Inherit: Inherit from 'Table data'  ExtrapMethod=Clip  InternalRulePriority=Speed  OutDataTypeStr=Inherit: Inherit via back propagation  RndMeth=Simplest  InputSameDT=off
  T : Outport
  wires:
  R/1 -> 1-D Lookup Table/1
  1-D Lookup Table/1 -> T/1

== system Sensor/SensorSub/Hex/CLHB03004_HexChange/FaltProcess ==
  T : Inport
  sClCddSensor_D_u8HvacEvapSensorErr : Inport  Port=2  OutDataTypeStr=uint8
  Switch : Switch  Criteria=u2 ~= 0  OutDataTypeStr=single  SaturateOnIntegerOverflow=off  InputSameDT=off
  Unit Delay : UnitDelay  SampleTime=-1  HasFrameUpgradeWarning=on
  sClCddSensor_Te_s32EvapRawValue : Outport  OutDataTypeStr=single
  wires:
  Unit Delay/1 -> Switch/1
  Switch/1 -> [sClCddSensor_Te_s32EvapRawValue], Unit Delay/1
  [T] -> Switch/3
  [sClCddSensor_D_u8HvacEvapSensorErr] -> Switch/2
  T/1 -> [T]
  sClCddSensor_D_u8HvacEvapSensorErr/1 -> [sClCddSensor_D_u8HvacEvapSensorErr]
  [sClCddSensor_Te_s32EvapRawValue] -> sClCddSensor_Te_s32EvapRawValue/1

== system Sensor/SensorSub/Hex/CLHB03004_HexChange/R2T ==
  R : Inport
  1-D Lookup Table : Lookup_n-D  NumberOfTableDimensions=1  BreakpointsForDimension1=tClCddSensor_Te_s32HexRtValue_X  BreakpointsForDimension1DataTypeStr=Inherit: Inherit from 'Breakpoint data'  Table=tClCddSensor_Te_s32HexRtValue  TableDataTypeStr=Inherit: Inherit from 'Table data'  ExtrapMethod=Clip  InternalRulePriority=Speed  OutDataTypeStr=Inherit: Inherit via back propagation  RndMeth=Simplest  InputSameDT=off
  T : Outport
  wires:
  R/1 -> 1-D Lookup Table/1
  1-D Lookup Table/1 -> T/1

== system Sensor/SensorSub/Hex/CLHB03004_HexChange/V2R ==
  V : Inport
  Bias : Bias  Bias=5  SaturateOnIntegerOverflow=off
  Divide : Product  Inputs=*/
  Gain : Gain  Gain=3000
  Gain1 : Gain  Gain=-1
  R : Outport
  wires:
  V/1 -> [V]
  [V] -> Gain1/1, Divide/1
  Gain1/1 -> Bias/1
  Bias/1 -> Divide/2
  Divide/1 -> Gain/1
  Gain/1 -> [R]
  [R] -> R/1

== system Sensor/SensorSub/InCar/CLHB03006_InCarChange/FaltProcess ==
  T : Inport
  "sClCddSensor_D_u8HvacIncarSensorErr  " : Inport  Port=2  OutDataTypeStr=uint8
  Switch : Switch  Criteria=u2 ~= 0  OutDataTypeStr=single  SaturateOnIntegerOverflow=off  InputSameDT=off
  Unit Delay : UnitDelay  SampleTime=-1  HasFrameUpgradeWarning=on
  sClCddSensor_Te_s32IncarRawValue : Outport  OutDataTypeStr=single
  wires:
  Unit Delay/1 -> Switch/1
  Switch/1 -> [sClCddSensor_Te_s32IncarRawValue], Unit Delay/1
  [T] -> Switch/3
  [sClCddSensor_D_u8HvacIncarSensorErr] -> Switch/2
  T/1 -> [T]
  "sClCddSensor_D_u8HvacIncarSensorErr  "/1 -> [sClCddSensor_D_u8HvacIncarSensorErr]
  [sClCddSensor_Te_s32IncarRawValue] -> sClCddSensor_Te_s32IncarRawValue/1

== system Sensor/SensorSub/InCar/CLHB03006_InCarChange/R2T ==
  R : Inport
  1-D Lookup Table : Lookup_n-D  NumberOfTableDimensions=1  BreakpointsForDimension1=tClCddSensor_Te_s32IncarRtValue_X  BreakpointsForDimension1DataTypeStr=Inherit: Inherit from 'Breakpoint data'  Table=tClCddSensor_Te_s32IncarRtValue  TableDataTypeStr=Inherit: Inherit from 'Table data'  ExtrapMethod=Clip  InternalRulePriority=Speed  OutDataTypeStr=Inherit: Inherit via back propagation  RndMeth=Simplest  InputSameDT=off
  T : Outport
  wires:
  R/1 -> 1-D Lookup Table/1
  1-D Lookup Table/1 -> T/1

== system Sensor/SensorSub/AQS/CLHB03007_AqsFlt/AqsInternalFlt/SigConfirm2 ==
  sigRaw : Inport
  Constant1 : Constant  Value=cClCddSensor_t_u8AQSErrorConfirm  OutDataTypeStr=uint8
  Constant2 : Constant  Value=cClCddSensor_t_u8AQSErrorRelieve  OutDataTypeStr=uint8
  SignalDelay1 : PCMULib/Standard/Relation&Logic/SignalDelay3
      settings: SourceProductName=PCMULib
  sig : Outport
  wires:
  [sigRaw] -> SignalDelay1/1
  Constant2/1 -> SignalDelay1/3
  SignalDelay1/1 -> [sig]
  Constant1/1 -> SignalDelay1/2
  sigRaw/1 -> [sigRaw]
  [sig] -> sig/1

== system Sensor/SensorSub/AQS/CLHB03007_AqsFlt/AqsPowerPinFlt/SigConfirm1 ==
  sigRaw : Inport
  Constant1 : Constant  Value=cClCddSensor_t_u8AQSErrorConfirm  OutDataTypeStr=uint8
  Constant2 : Constant  Value=cClCddSensor_t_u8AQSErrorRelieve  OutDataTypeStr=uint8
  SignalDelay1 : PCMULib/Standard/Relation&Logic/SignalDelay3
      settings: SourceProductName=PCMULib
  sig : Outport
  wires:
  [sig] -> sig/1
  sigRaw/1 -> [sigRaw]
  Constant1/1 -> SignalDelay1/2
  SignalDelay1/1 -> [sig]
  Constant2/1 -> SignalDelay1/3
  [sigRaw] -> SignalDelay1/1

== system Sensor/SensorSub/AQS/CLHB03007_AqsFlt/PWMDetPinFlt/SigConfirm ==
  sigRaw : Inport
  Constant1 : Constant  Value=cClCddSensor_t_u8AQSErrorConfirm  OutDataTypeStr=uint8
  Constant2 : Constant  Value=cClCddSensor_t_u8AQSErrorRelieve  OutDataTypeStr=uint8
  SignalDelay1 : PCMULib/Standard/Relation&Logic/SignalDelay3
      settings: SourceProductName=PCMULib
  sig : Outport
  wires:
  [sigRaw] -> SignalDelay1/1
  Constant2/1 -> SignalDelay1/3
  SignalDelay1/1 -> [sig]
  Constant1/1 -> SignalDelay1/2
  sigRaw/1 -> [sigRaw]
  [sig] -> sig/1
